simulink model "dc_motor_model_basic_blocks_current_control"  (R2014a)
settings: Solver=ode15s  StartTime=0.0  StopTime=10.0  FixedStep=0.001  MinStep=0.001  RelTol=1e-3
values from neighbouring files (symbols this model uses):
  I_d = 0.2    [dc_motor_basic_blocks_current_control.m]
  J = 8.85*10^(-7)    (= 8.85e-07)    [dc_motor_basic_blocks_current_control.m]
  k_emf = k_tau    (= 0.0452)    [dc_motor_basic_blocks_current_control.m]
  k_tau = 0.0452    [dc_motor_basic_blocks_current_control.m]
  Kd = 0    [dc_motor_basic_blocks_current_control.m]
  Ki = 100    [dc_motor_basic_blocks_current_control.m]
  Kp = 10    [dc_motor_basic_blocks_current_control.m]
  L = 0.746*10^(-3)    (= 0.000746)    [dc_motor_basic_blocks_current_control.m]
  mu = 10^(-6)    (= 1e-06)    [dc_motor_basic_blocks_current_control.m]
  R = 7.25    [dc_motor_basic_blocks_current_control.m]
  t0 = 0.1    [dc_motor_basic_blocks_current_control.m]
  T_load = 0.001    [dc_motor_basic_blocks_current_control.m]
  V_MAX = 24    [dc_motor_basic_blocks_current_control.m]
libraries: simulink x1
settings Model: Creator=krzysztof  LastModifiedBy=krzysztof
settings DataIOCC: SignalLoggingSaveFormat=ModelDataLogs
settings OptimizationCC: ExpressionDepthLimit=2147483647
settings DebuggingCC: UnderspecifiedInitializationDetection=Classic  FcnCallInpInsideContextMsg=EnableAllAsWarning  StateNameClashWarn=warning
settings GRTTargetCC: CombineOutputUpdateFcns=off  GRTInterface=on

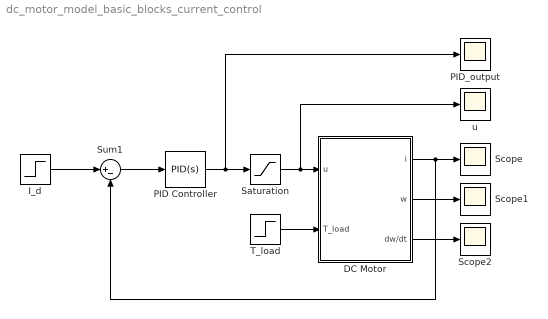
== system dc_motor_model_basic_blocks_current_control ==
  DC Motor : Subsystem
  I_d : Step  Time=t0  After=I_d  SampleTime=0
  PID Controller : simulink/Continuous/PID Controller  Controller=PID  TimeDomain=Continuous-time  SampleTime=1  IntegratorMethod=Forward Euler  FilterMethod=Forward Euler  Form=Parallel  P=Kp  I=Ki  D=Kd  N=100  InitialConditionSource=internal  InitialConditionForIntegrator=0  InitialConditionForFilter=0  ExternalReset=none  LimitOutput=off  UpperSaturationLimit=inf  LowerSaturationLimit=-inf  LinearizeAsGain=off  AntiWindupMode=none  Kb=1  TrackingMode=off  Kt=1  PParamMin=[]  PParamMax=[]  IParamMin=[]  IParamMax=[]  DParamMin=[]  DParamMax=[]  NParamMin=[]  NParamMax=[]  KbParamMin=[]  KbParamMax=[]  KtParamMin=[]  KtParamMax=[]  POutMin=[]  POutMax=[]  IOutMin=[]  IOutMax=[]  DOutMin=[]  DOutMax=[]  NOutMin=[]  NOutMax=[]  KbOutMin=[]  KbOutMax=[]  KtOutMin=[]  KtOutMax=[]  IntegratorOutMin=[]  IntegratorOutMax=[]  FilterOutMin=[]  FilterOutMax=[]  SumOutMin=[]  SumOutMax=[]  SumI1OutMin=[]  SumI1OutMax=[]  SumI2OutMin=[]  SumI2OutMax=[]  SumI3OutMin=[]  SumI3OutMax=[]  SumDOutMin=[]  SumDOutMax=[]  SaturationOutMin=[]  SaturationOutMax=[]  IntegratorContinuousStateAttributes=''  IntegratorStateMustResolveToSignalObject=off  IntegratorRTWStateStorageClass=Auto  FilterContinuousStateAttributes=''  FilterStateMustResolveToSignalObject=off  FilterRTWStateStorageClass=Auto
  "PID_output " : Scope
      settings: SaveName=pid_out
  Saturation : Saturate  UpperLimit=V_MAX  LowerLimit=0
  Scope : Scope
      settings: SaveName=i_motor
  Scope1 : Scope
      settings: SaveName=w
  Scope2 : Scope
  Sum1 : Sum  Inputs=|+-
  "T_load " : Step  Time=t0  After=T_load  SampleTime=0
  u : Scope
      settings: SaveName=u_input
  wires:
  "T_load "/1 -> DC Motor/2(T_load)
  DC Motor/1(i) -> Scope/1, Sum1/2
  DC Motor/3(dw/dt) -> Scope2/1
  DC Motor/2(w) -> Scope1/1
  I_d/1 -> Sum1/1
  Sum1/1 -> PID Controller/1
  Saturation/1 -> u/1, DC Motor/1(u)
  PID Controller/1 -> "PID_output "/1, Saturation/1

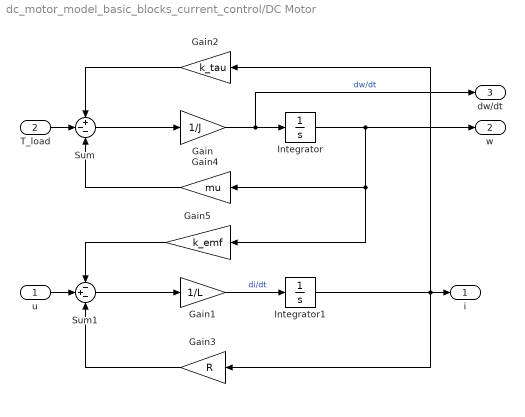
== system dc_motor_model_basic_blocks_current_control/DC Motor ==
  u : Inport
  T_load : Inport  Port=2
  Gain : Gain  Gain=1/J
  Gain1 : Gain  Gain=1/L
  Gain2 : Gain  Gain=k_tau
  Gain3 : Gain  Gain=R
  Gain4 : Gain  Gain=mu
  Gain5 : Gain  Gain=k_emf
  Integrator : Integrator
  Integrator1 : Integrator
  Sum : Sum  Inputs=+--
  Sum1 : Sum  Inputs=-+-
  i : Outport
  w : Outport  Port=2
  dw/dt : Outport  Port=3
  wires:
  Integrator/1 -> Gain4/1, Gain5/1, w/1
  Integrator1/1 -> Gain2/1, Gain3/1, i/1
  Gain/1 -> Integrator/1, dw/dt/1  "dw/dt"
  Gain1/1 -> Integrator1/1  "di/dt"
  Sum/1 -> Gain/1
  Sum1/1 -> Gain1/1
  Gain2/1 -> Sum/1
  Gain3/1 -> Sum1/3
  Gain4/1 -> Sum/3
  Gain5/1 -> Sum1/1
  T_load/1 -> Sum/2
  u/1 -> Sum1/2
